simulink model "Exercise4Pt2Easier"  (R2019b)
settings: Solver=VariableStepAuto  StartTime=0.0  StopTime=10.0  RelTol=1e-3
values from neighbouring files (symbols this model uses):
  a_in = 0    [NewtonsSecondLaw.m]
  c = 16    [NewtonsSecondLaw.m]
  Q_in = (10*0.134)/60    (= 0.0223333333333)    [NewtonsSecondLaw.m]
settings Model: Creator=dzecc  LastModifiedBy=dzecc

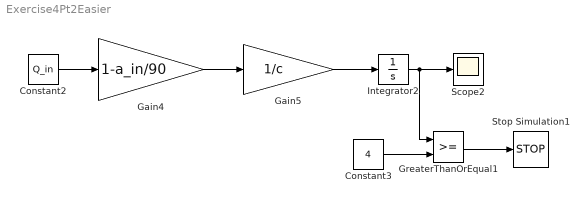
== system Exercise4Pt2Easier ==
  Constant2 : Constant  Value=Q_in  VectorParams1D=off  SampleTime=10
  Constant3 : Constant  Value=4  SampleTime=10
  Gain4 : Gain  Gain=1-a_in/90
  Gain5 : Gain  Gain=1/c
  GreaterThanOrEqual1 : RelationalOperator  OutDataTypeStr=boolean  RndMeth=Simplest
  Integrator2 : Integrator
  Scope2 : Scope
  Stop Simulation1 : Stop
  wires:
  Constant2/1 -> Gain4/1
  Gain4/1 -> Gain5/1
  GreaterThanOrEqual1/1 -> Stop Simulation1/1
  Integrator2/1 -> GreaterThanOrEqual1/1, Scope2/1
  Constant3/1 -> GreaterThanOrEqual1/2
  Gain5/1 -> Integrator2/1
